simulink model "prova_controllo_motore"  (R2013a)
settings: Solver=ode1  StartTime=0.0  StopTime=9  FixedStep=0.001  RelTol=1e-3
undefined symbols (not defined in the file or in its folder): sigbuilder_block
libraries: qbmove_library x2, QB_pacer_lib x1, simulink x1
settings Model: Creator=laurentio  LastModifiedBy=laurentio

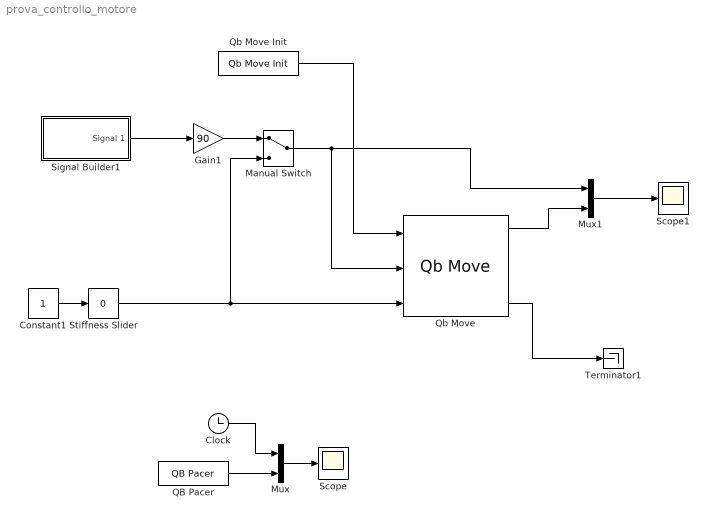
== system prova_controllo_motore ==
  Clock : Clock
  Constant1 : Constant
  Gain1 : Gain  Gain=90
  Manual Switch : ManualSwitch
  Mux : Mux  Inputs=2
  Mux1 : Mux  Inputs=2
  QB Pacer : QB_pacer_lib/QB Pacer  simTimePerRealTime=1
  Qb Move : qbmove_library/Qb Move  ID=48  ACTIVE_COMM_DIRECTIONS=Both  CONTROL_MODE=Equilibrium Position and Stiffness Preset  DAISY_CHAINING=off  MAX_ANG=0  SW_LIMIT=inf  OFFSET=0
  Qb Move Init : qbmove_library/Qb Move Init  NUMBER_OF_COM='/dev/tty.usbserial-48'
  Scope : Scope
      settings: YMin=0  YMax=5.5
  Scope1 : Scope
      settings: YMax=95
  Signal Builder1 : Subsystem  Tag=STV Subsys  LoadFcn=sigbuilder_block('load');  StartFcn=sigbuilder_block('start');  StopFcn=sigbuilder_block('stop');  ClipboardFcn=sigbuilder_block('clipboard');  mask(Sigbuilder block){}
      mask help: Simulink:masks:SigbuilderBlock_MD
      mask init:
      | if ~strcmp(get_param(bdroot(gcbh),'SimulationStatus'),'stopped') tuvar = sigbuilder_block('maskInit'); end
      settings: CopyFcn=sigbuilder_block('copy');  DeleteFcn=sigbuilder_block('delete');  ModelCloseFcn=sigbuilder_block('modelClose');  PreSaveFcn=sigbuilder_block('preSave');  PauseFcn=sigbuilder_block('pause');  ContinueFcn=sigbuilder_block('continue');  NameChangeFcn=sigbuilder_block('namechange');  OpenFcn=sigbuilder_block('open',[-1537.68 106.631 1436.04 660.716 ]);  CloseFcn=sigbuilder_block('close');
      mask Display: plot(0, 0, 100, 100,[2, 2, 32, 32, 2], [68, 8, 8, 68, 68],[32, 2], [38, 38], [32, 19, 2],[53, 60, 44], [32, 17, 17, 2],[16, 16, 31, 31]);txt = getActiveGroup(gcbh);text(2, 100, txt,'verticalAlignment', 'top');
  Stiffness Slider : simulink/Math Operations/Slider Gain  low=0  gain=0  high=30
  Terminator1 : Terminator
  wires:
  Qb Move Init/1 -> Qb Move/1
  Constant1/1 -> Stiffness Slider/1
  Stiffness Slider/1 -> Manual Switch/2, Qb Move/3
  QB Pacer/1 -> Mux/2
  Qb Move/4 -> Terminator1/1
  Clock/1 -> Mux/1
  Mux/1 -> Scope/1
  Mux1/1 -> Scope1/1
  Qb Move/1 -> Mux1/2
  Signal Builder1/1(Signal 1) -> Gain1/1
  Gain1/1 -> Manual Switch/1
  Manual Switch/1 -> Qb Move/2, Mux1/1

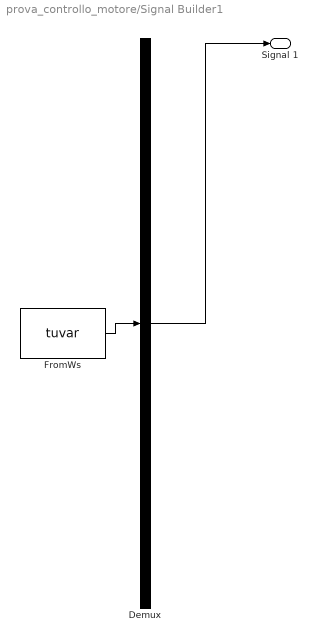
== system prova_controllo_motore/Signal Builder1 ==
  Demux : Demux  Tag=STV Demux  Outputs=1
  FromWs : FromWorkspace  Tag=STV FromWs  VariableName=tuvar  SampleTime=0
      SigBuilderData=|
      | common.afterFinalStr = 'Extrapolate'
      | common.sampleTime = 0
      | dataSet.timeRange = [0 9]
      | dataSet.name = 'Group 1'
      | sbobj.Groups.Name = 'Group 1'
      | sbobj.Groups.Signals.Name = 'Signal 1'
      | sbobj.Groups.Signals.XData = [0 1 1 2 2 3 3 4 4 5 5 6 6 7 7 8 8 9]
      | sbobj.Groups.Signals.YData = [0 0 1 1 0 0 1 1 0 0 1 1 0 0 1 1 0 0]
      | sbobj.Groups.TimeRange = [0 9]
  Signal 1 : Outport  Tag=STV Outport
  wires:
  FromWs/1 -> Demux/1
  Demux/1 -> Signal 1/1
